simulink model "coif2_7_Level"  (R2021a)
settings: Solver=VariableStepAuto  StartTime=0.0  StopTime=8  RelTol=1e-3
undefined symbols (not defined in the file): lambda2
libraries: dspsigops x15, dspquant2 x1
(part 2 of 4)

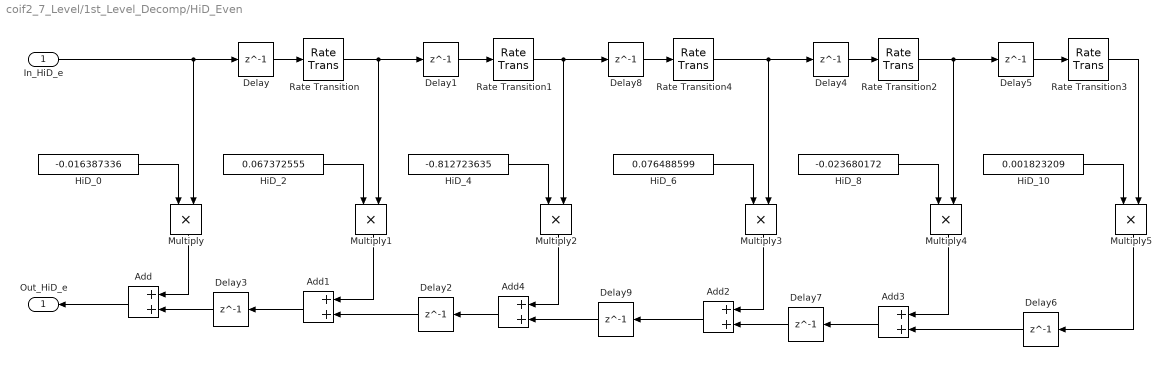
== system coif2_7_Level/1st_Level_Decomp/HiD_Even ==
  In_HiD_e : Inport  OutDataTypeStr=double  SampleTime=1/44100
  Add{,1..4} (5 alike) : Sum  AccumDataTypeStr=double  OutDataTypeStr=double
  Delay{,1..9} (10 alike) : Delay  DelayLength=1  SampleTime=1/44100
  HiD_0 : Constant  Value=-0.016387336  OutDataTypeStr=double  SampleTime=1/44100
  HiD_10 : Constant  Value=0.001823209  OutDataTypeStr=double  SampleTime=1/44100
  HiD_2 : Constant  Value=0.067372555  OutDataTypeStr=double  SampleTime=1/44100
  HiD_4 : Constant  Value=-0.812723635  OutDataTypeStr=double  SampleTime=1/44100
  HiD_6 : Constant  Value=0.076488599  OutDataTypeStr=double  SampleTime=1/44100
  HiD_8 : Constant  Value=-0.023680172  OutDataTypeStr=double  SampleTime=1/44100
  Multiply{,1..5} (6 alike) : Product  OutDataTypeStr=double
  Rate Transition{,1..4} (5 alike) : RateTransition  OutPortSampleTime=1/44100
  Out_HiD_e : Outport  OutDataTypeStr=double  SampleTime=1/44100  VectorParamsAs1DForOutWhenUnconnected=off
  wires:
  In_HiD_e/1 -> Delay/1, Multiply/2
  Delay3/1 -> Add/2
  HiD_2/1 -> Multiply1/1
  Delay/1 -> Rate Transition/1
  Multiply/1 -> Add/1
  Rate Transition/1 -> Delay1/1, Multiply1/2
  HiD_4/1 -> Multiply2/1
  Delay2/1 -> Add1/2
  Multiply1/1 -> Add1/1
  Add1/1 -> Delay3/1
  Rate Transition1/1 -> Delay8/1, Multiply2/2
  Add/1 -> Out_HiD_e/1
  Delay1/1 -> Rate Transition1/1
  HiD_0/1 -> Multiply/1
  HiD_6/1 -> Multiply3/1
  Delay7/1 -> Add2/2
  Delay5/1 -> Rate Transition3/1
  Rate Transition3/1 -> Multiply5/2
  Add3/1 -> Delay7/1
  Multiply3/1 -> Add2/1
  Rate Transition2/1 -> Delay5/1, Multiply4/2
  Delay6/1 -> Add3/2
  Multiply4/1 -> Add3/1
  Multiply5/1 -> Delay6/1
  HiD_10/1 -> Multiply5/1
  Delay4/1 -> Rate Transition2/1
  HiD_8/1 -> Multiply4/1
  Delay8/1 -> Rate Transition4/1
  Rate Transition4/1 -> Multiply3/2, Delay4/1
  Add2/1 -> Delay9/1
  Multiply2/1 -> Add4/1
  Add4/1 -> Delay2/1
  Delay9/1 -> Add4/2

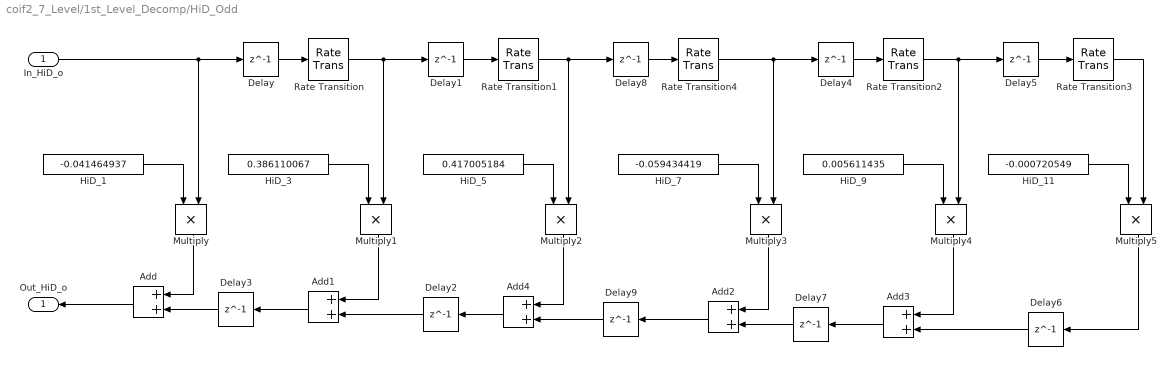
== system coif2_7_Level/1st_Level_Decomp/HiD_Odd ==
  In_HiD_o : Inport  OutDataTypeStr=double  SampleTime=1/44100
  Add{,1..4} (5 alike) : Sum  AccumDataTypeStr=double  OutDataTypeStr=double
  Delay{,1..9} (10 alike) : Delay  DelayLength=1  SampleTime=1/44100
  HiD_1 : Constant  Value=-0.041464937  OutDataTypeStr=double  SampleTime=1/44100
  HiD_11 : Constant  Value=-0.000720549  OutDataTypeStr=double  SampleTime=1/44100
  HiD_3 : Constant  Value=0.386110067  OutDataTypeStr=double  SampleTime=1/44100
  HiD_5 : Constant  Value=0.417005184  OutDataTypeStr=double  SampleTime=1/44100
  HiD_7 : Constant  Value=-0.059434419  OutDataTypeStr=double  SampleTime=1/44100
  HiD_9 : Constant  Value=0.005611435  OutDataTypeStr=double  SampleTime=1/44100
  Multiply{,1..5} (6 alike) : Product  OutDataTypeStr=double
  Rate Transition{,1..4} (5 alike) : RateTransition  OutPortSampleTime=1/44100
  Out_HiD_o : Outport  OutDataTypeStr=double  SampleTime=1/44100  VectorParamsAs1DForOutWhenUnconnected=off
  wires:
  Add/1 -> Out_HiD_o/1
  Add4/1 -> Delay2/1
  Delay8/1 -> Rate Transition4/1
  Rate Transition4/1 -> Multiply3/2, Delay4/1
  HiD_7/1 -> Multiply3/1
  Add2/1 -> Delay9/1
  Delay1/1 -> Rate Transition1/1
  Delay2/1 -> Add1/2
  Delay6/1 -> Add3/2
  HiD_9/1 -> Multiply4/1
  Add3/1 -> Delay7/1
  Multiply3/1 -> Add2/1
  Multiply5/1 -> Delay6/1
  Delay7/1 -> Add2/2
  HiD_3/1 -> Multiply1/1
  Multiply4/1 -> Add3/1
  Rate Transition3/1 -> Multiply5/2
  HiD_1/1 -> Multiply/1
  HiD_11/1 -> Multiply5/1
  Delay4/1 -> Rate Transition2/1
  Rate Transition2/1 -> Delay5/1, Multiply4/2
  Multiply2/1 -> Add4/1
  Delay/1 -> Rate Transition/1
  Rate Transition/1 -> Delay1/1, Multiply1/2
  Delay5/1 -> Rate Transition3/1
  Delay9/1 -> Add4/2
  Multiply1/1 -> Add1/1
  Rate Transition1/1 -> Delay8/1, Multiply2/2
  Multiply/1 -> Add/1
  Add1/1 -> Delay3/1
  Delay3/1 -> Add/2
  In_HiD_o/1 -> Delay/1, Multiply/2
  HiD_5/1 -> Multiply2/1

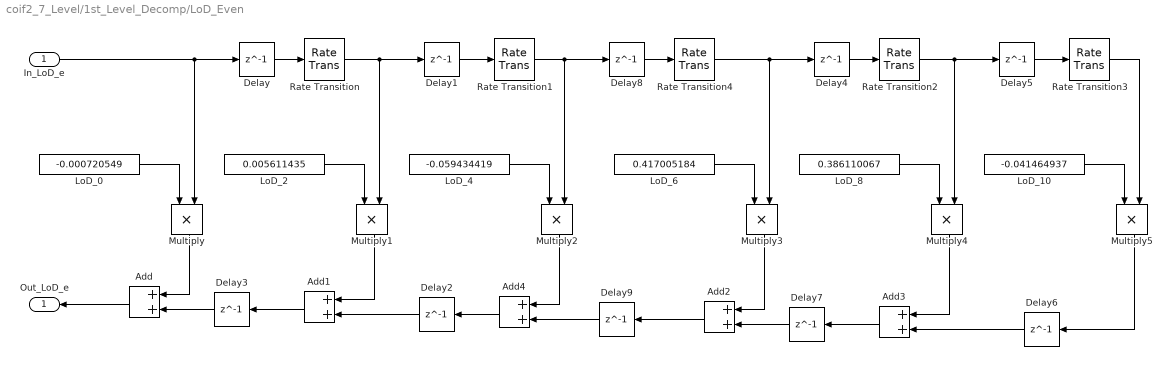
== system coif2_7_Level/1st_Level_Decomp/LoD_Even ==
  In_LoD_e : Inport  OutDataTypeStr=double  SampleTime=1/44100
  Add{,1..4} (5 alike) : Sum  AccumDataTypeStr=double  OutDataTypeStr=double
  Delay{,1..9} (10 alike) : Delay  DelayLength=1  SampleTime=1/44100
  LoD_0 : Constant  Value=-0.000720549  OutDataTypeStr=double  SampleTime=1/44100
  LoD_10 : Constant  Value=-0.041464937  OutDataTypeStr=double  SampleTime=1/44100
  LoD_2 : Constant  Value=0.005611435  OutDataTypeStr=double  SampleTime=1/44100
  LoD_4 : Constant  Value=-0.059434419  OutDataTypeStr=double  SampleTime=1/44100
  LoD_6 : Constant  Value=0.417005184  OutDataTypeStr=double  SampleTime=1/44100
  LoD_8 : Constant  Value=0.386110067  OutDataTypeStr=double  SampleTime=1/44100
  Multiply{,1..5} (6 alike) : Product  OutDataTypeStr=double
  Rate Transition{,1..4} (5 alike) : RateTransition  OutPortSampleTime=1/44100
  Out_LoD_e : Outport  OutDataTypeStr=double  SampleTime=1/44100  VectorParamsAs1DForOutWhenUnconnected=off
  wires:
  Delay3/1 -> Add/2
  Rate Transition1/1 -> Delay8/1, Multiply2/2
  Add/1 -> Out_LoD_e/1
  Add1/1 -> Delay3/1
  Multiply/1 -> Add/1
  In_LoD_e/1 -> Delay/1, Multiply/2
  Rate Transition/1 -> Delay1/1, Multiply1/2
  LoD_4/1 -> Multiply2/1
  Delay/1 -> Rate Transition/1
  Delay9/1 -> Add4/2
  Multiply1/1 -> Add1/1
  Multiply2/1 -> Add4/1
  LoD_2/1 -> Multiply1/1
  Delay4/1 -> Rate Transition2/1
  Multiply5/1 -> Delay6/1
  Multiply4/1 -> Add3/1
  Rate Transition2/1 -> Delay5/1, Multiply4/2
  LoD_10/1 -> Multiply5/1
  Delay2/1 -> Add1/2
  Delay5/1 -> Rate Transition3/1
  Multiply3/1 -> Add2/1
  LoD_8/1 -> Multiply4/1
  Delay7/1 -> Add2/2
  Rate Transition3/1 -> Multiply5/2
  Delay6/1 -> Add3/2
  Add3/1 -> Delay7/1
  LoD_6/1 -> Multiply3/1
  LoD_0/1 -> Multiply/1
  Add2/1 -> Delay9/1
  Delay8/1 -> Rate Transition4/1
  Rate Transition4/1 -> Multiply3/2, Delay4/1
  Delay1/1 -> Rate Transition1/1
  Add4/1 -> Delay2/1

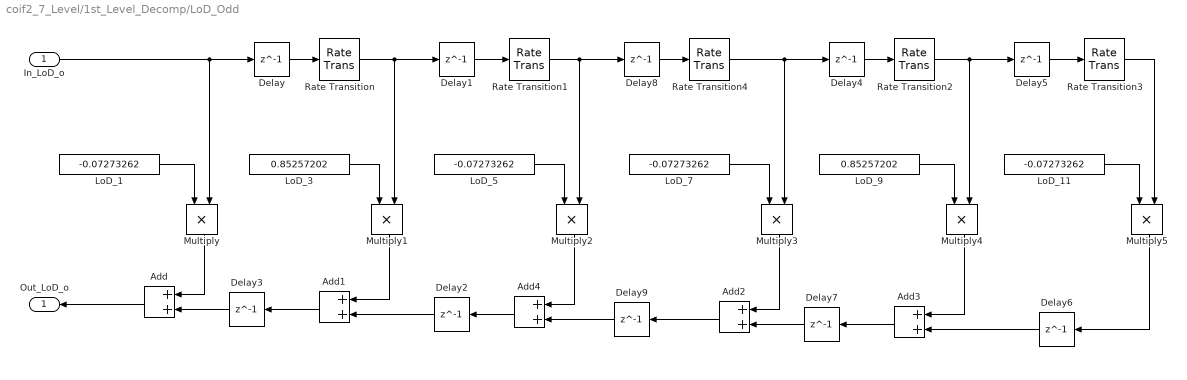
== system coif2_7_Level/1st_Level_Decomp/LoD_Odd ==
  In_LoD_o : Inport  OutDataTypeStr=double  SampleTime=1/44100
  Add{,1..4} (5 alike) : Sum  AccumDataTypeStr=double  OutDataTypeStr=double
  Delay{,1..9} (10 alike) : Delay  DelayLength=1  SampleTime=1/44100
  LoD_{1,5,7,11} (4 alike) : Constant  Value=-0.07273262  OutDataTypeStr=double  SampleTime=1/44100
  LoD_3 : Constant  Value=0.85257202  OutDataTypeStr=double  SampleTime=1/44100
  LoD_9 : Constant  Value=0.85257202  OutDataTypeStr=double  SampleTime=1/44100
  Multiply{,1..5} (6 alike) : Product  OutDataTypeStr=double
  Rate Transition{,1..4} (5 alike) : RateTransition  OutPortSampleTime=1/44100
  Out_LoD_o : Outport  OutDataTypeStr=double  SampleTime=1/44100  VectorParamsAs1DForOutWhenUnconnected=off
  wires:
  LoD_9/1 -> Multiply4/1
  Add3/1 -> Delay7/1
  Rate Transition4/1 -> Multiply3/2, Delay4/1
  Delay2/1 -> Add1/2
  Delay1/1 -> Rate Transition1/1
  Delay8/1 -> Rate Transition4/1
  LoD_5/1 -> Multiply2/1
  Add4/1 -> Delay2/1
  LoD_11/1 -> Multiply5/1
  LoD_1/1 -> Multiply/1
  Multiply3/1 -> Add2/1
  LoD_3/1 -> Multiply1/1
  In_LoD_o/1 -> Delay/1, Multiply/2
  Add/1 -> Out_LoD_o/1
  Rate Transition1/1 -> Delay8/1, Multiply2/2
  Multiply1/1 -> Add1/1
  Delay/1 -> Rate Transition/1
  Rate Transition/1 -> Delay1/1, Multiply1/2
  Multiply2/1 -> Add4/1
  LoD_7/1 -> Multiply3/1
  Rate Transition2/1 -> Delay5/1, Multiply4/2
  Delay4/1 -> Rate Transition2/1
  Multiply5/1 -> Delay6/1
  Delay7/1 -> Add2/2
  Rate Transition3/1 -> Multiply5/2
  Delay3/1 -> Add/2
  Delay5/1 -> Rate Transition3/1
  Add2/1 -> Delay9/1
  Add1/1 -> Delay3/1
  Delay9/1 -> Add4/2
  Delay6/1 -> Add3/2
  Multiply4/1 -> Add3/1
  Multiply/1 -> Add/1

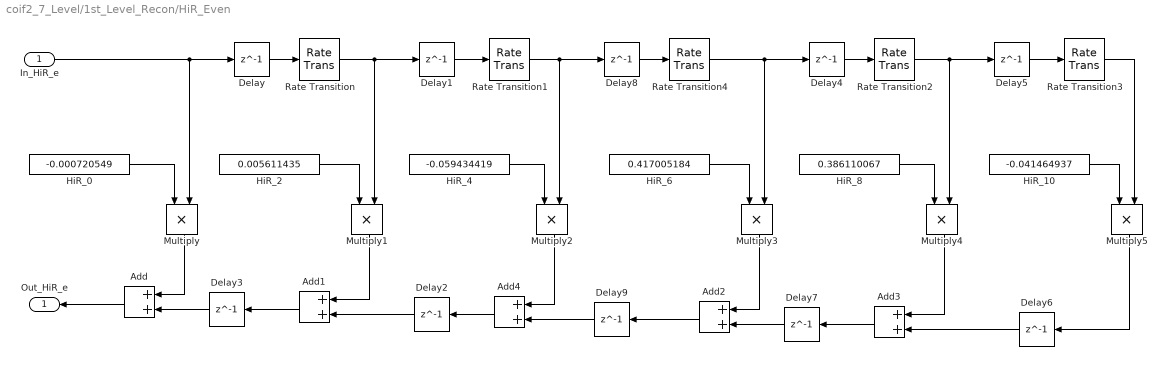
== system coif2_7_Level/1st_Level_Recon/HiR_Even ==
  In_HiR_e : Inport  OutDataTypeStr=double  SampleTime=1/44100
  Add{,1..4} (5 alike) : Sum  AccumDataTypeStr=double  OutDataTypeStr=double
  Delay{,1..9} (10 alike) : Delay  DelayLength=1  SampleTime=1/44100
  HiR_0 : Constant  Value=-0.000720549  OutDataTypeStr=double  SampleTime=1/44100
  HiR_10 : Constant  Value=-0.041464937  OutDataTypeStr=double  SampleTime=1/44100
  HiR_2 : Constant  Value=0.005611435  OutDataTypeStr=double  SampleTime=1/44100
  HiR_4 : Constant  Value=-0.059434419  OutDataTypeStr=double  SampleTime=1/44100
  HiR_6 : Constant  Value=0.417005184  OutDataTypeStr=double  SampleTime=1/44100
  HiR_8 : Constant  Value=0.386110067  OutDataTypeStr=double  SampleTime=1/44100
  Multiply{,1..5} (6 alike) : Product  OutDataTypeStr=double
  Rate Transition{,1..4} (5 alike) : RateTransition  OutPortSampleTime=1/44100
  Out_HiR_e : Outport  OutDataTypeStr=double  SampleTime=1/44100  VectorParamsAs1DForOutWhenUnconnected=off
  wires:
  Multiply1/1 -> Add1/1
  Delay4/1 -> Rate Transition2/1
  Add4/1 -> Delay2/1
  Delay9/1 -> Add4/2
  Rate Transition4/1 -> Multiply3/2, Delay4/1
  Rate Transition3/1 -> Multiply5/2
  Add1/1 -> Delay3/1
  Add3/1 -> Delay7/1
  Delay8/1 -> Rate Transition4/1
  Multiply5/1 -> Delay6/1
  Add2/1 -> Delay9/1
  Multiply4/1 -> Add3/1
  HiR_8/1 -> Multiply4/1
  Delay6/1 -> Add3/2
  Rate Transition1/1 -> Delay8/1, Multiply2/2
  In_HiR_e/1 -> Delay/1, Multiply/2
  HiR_0/1 -> Multiply/1
  Multiply2/1 -> Add4/1
  Delay7/1 -> Add2/2
  Rate Transition2/1 -> Delay5/1, Multiply4/2
  Add/1 -> Out_HiR_e/1
  Multiply3/1 -> Add2/1
  HiR_6/1 -> Multiply3/1
  Multiply/1 -> Add/1
  HiR_4/1 -> Multiply2/1
  Delay2/1 -> Add1/2
  Delay5/1 -> Rate Transition3/1
  Delay3/1 -> Add/2
  Delay1/1 -> Rate Transition1/1
  HiR_2/1 -> Multiply1/1
  Rate Transition/1 -> Delay1/1, Multiply1/2
  Delay/1 -> Rate Transition/1
  HiR_10/1 -> Multiply5/1

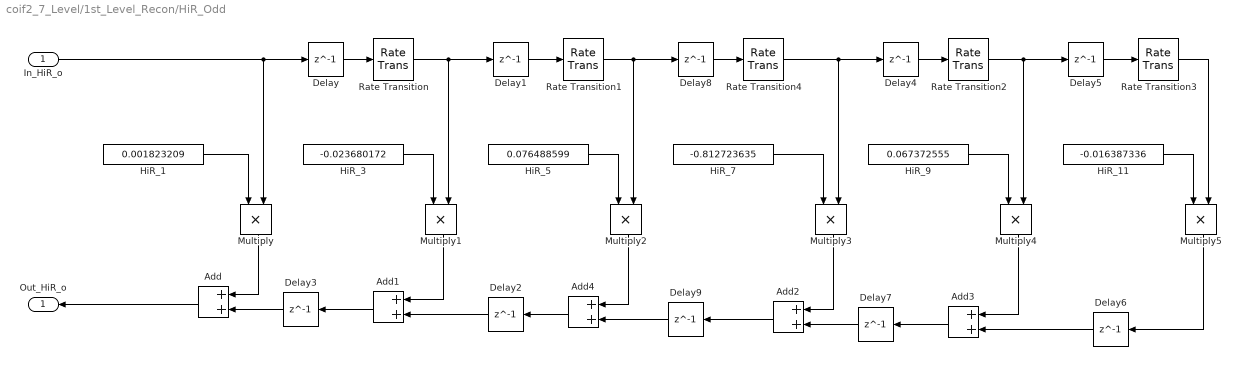
== system coif2_7_Level/1st_Level_Recon/HiR_Odd ==
  In_HiR_o : Inport  OutDataTypeStr=double  SampleTime=1/44100
  Add{,1..4} (5 alike) : Sum  AccumDataTypeStr=double  OutDataTypeStr=double
  Delay{,1..9} (10 alike) : Delay  DelayLength=1  SampleTime=1/44100
  HiR_1 : Constant  Value=0.001823209  OutDataTypeStr=double  SampleTime=1/44100
  HiR_11 : Constant  Value=-0.016387336  OutDataTypeStr=double  SampleTime=1/44100
  HiR_3 : Constant  Value=-0.023680172  OutDataTypeStr=double  SampleTime=1/44100
  HiR_5 : Constant  Value=0.076488599  OutDataTypeStr=double  SampleTime=1/44100
  HiR_7 : Constant  Value=-0.812723635  OutDataTypeStr=double  SampleTime=1/44100
  HiR_9 : Constant  Value=0.067372555  OutDataTypeStr=double  SampleTime=1/44100
  Multiply{,1..5} (6 alike) : Product  OutDataTypeStr=double
  Rate Transition{,1..4} (5 alike) : RateTransition  OutPortSampleTime=1/44100
  Out_HiR_o : Outport  OutDataTypeStr=double  SampleTime=1/44100  VectorParamsAs1DForOutWhenUnconnected=off
  wires:
  HiR_9/1 -> Multiply4/1
  Add2/1 -> Delay9/1
  Rate Transition/1 -> Delay1/1, Multiply1/2
  HiR_7/1 -> Multiply3/1
  Multiply2/1 -> Add4/1
  Rate Transition2/1 -> Delay5/1, Multiply4/2
  Rate Transition4/1 -> Multiply3/2, Delay4/1
  HiR_5/1 -> Multiply2/1
  Multiply5/1 -> Delay6/1
  HiR_11/1 -> Multiply5/1
  Multiply1/1 -> Add1/1
  Delay5/1 -> Rate Transition3/1
  Add1/1 -> Delay3/1
  Multiply/1 -> Add/1
  Delay7/1 -> Add2/2
  Delay2/1 -> Add1/2
  Delay9/1 -> Add4/2
  Delay4/1 -> Rate Transition2/1
  Delay3/1 -> Add/2
  Multiply3/1 -> Add2/1
  Delay8/1 -> Rate Transition4/1
  Rate Transition3/1 -> Multiply5/2
  Delay1/1 -> Rate Transition1/1
  Delay6/1 -> Add3/2
  Add4/1 -> Delay2/1
  Rate Transition1/1 -> Delay8/1, Multiply2/2
  Add/1 -> Out_HiR_o/1
  Add3/1 -> Delay7/1
  HiR_3/1 -> Multiply1/1
  In_HiR_o/1 -> Multiply/2, Delay/1
  Delay/1 -> Rate Transition/1
  HiR_1/1 -> Multiply/1
  Multiply4/1 -> Add3/1

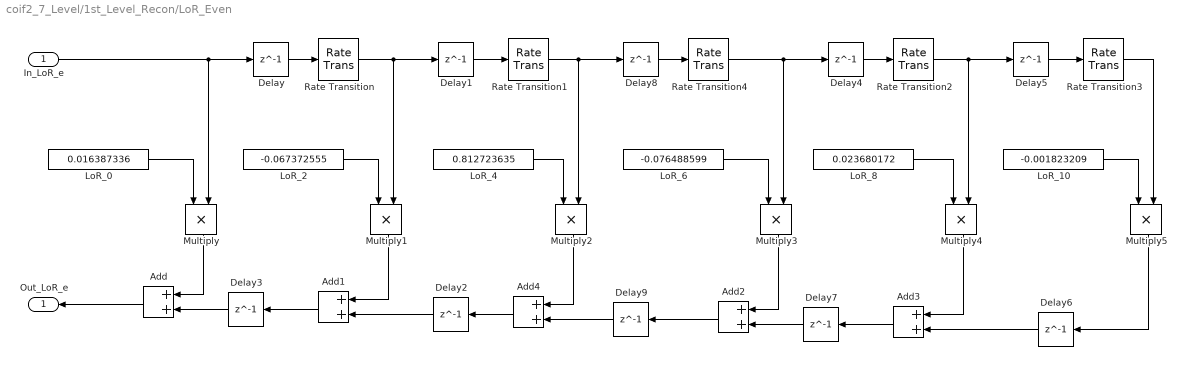
== system coif2_7_Level/1st_Level_Recon/LoR_Even ==
  In_LoR_e : Inport  OutDataTypeStr=double  SampleTime=1/44100
  Add{,1..4} (5 alike) : Sum  AccumDataTypeStr=double  OutDataTypeStr=double
  Delay{,1..9} (10 alike) : Delay  DelayLength=1  SampleTime=1/44100
  LoR_0 : Constant  Value=0.016387336  OutDataTypeStr=double  SampleTime=1/44100
  LoR_10 : Constant  Value=-0.001823209  OutDataTypeStr=double  SampleTime=1/44100
  LoR_2 : Constant  Value=-0.067372555  OutDataTypeStr=double  SampleTime=1/44100
  LoR_4 : Constant  Value=0.812723635  OutDataTypeStr=double  SampleTime=1/44100
  LoR_6 : Constant  Value=-0.076488599  OutDataTypeStr=double  SampleTime=1/44100
  LoR_8 : Constant  Value=0.023680172  OutDataTypeStr=double  SampleTime=1/44100
  Multiply{,1..5} (6 alike) : Product  OutDataTypeStr=double
  Rate Transition{,1..4} (5 alike) : RateTransition  OutPortSampleTime=1/44100
  Out_LoR_e : Outport  OutDataTypeStr=double  SampleTime=1/44100  VectorParamsAs1DForOutWhenUnconnected=off
  wires:
  LoR_4/1 -> Multiply2/1
  LoR_10/1 -> Multiply5/1
  LoR_8/1 -> Multiply4/1
  LoR_0/1 -> Multiply/1
  LoR_2/1 -> Multiply1/1
  Add2/1 -> Delay9/1
  In_LoR_e/1 -> Multiply/2, Delay/1
  Multiply4/1 -> Add3/1
  Delay8/1 -> Rate Transition4/1
  Add3/1 -> Delay7/1
  Rate Transition3/1 -> Multiply5/2
  Add4/1 -> Delay2/1
  Delay4/1 -> Rate Transition2/1
  Multiply1/1 -> Add1/1
  Delay5/1 -> Rate Transition3/1
  Delay2/1 -> Add1/2
  Delay3/1 -> Add/2
  Delay1/1 -> Rate Transition1/1
  Multiply/1 -> Add/1
  Multiply3/1 -> Add2/1
  Delay9/1 -> Add4/2
  Rate Transition2/1 -> Delay5/1, Multiply4/2
  Rate Transition4/1 -> Multiply3/2, Delay4/1
  Add1/1 -> Delay3/1
  LoR_6/1 -> Multiply3/1
  Multiply5/1 -> Delay6/1
  Add/1 -> Out_LoR_e/1
  Rate Transition1/1 -> Delay8/1, Multiply2/2
  Delay6/1 -> Add3/2
  Multiply2/1 -> Add4/1
  Delay7/1 -> Add2/2
  Rate Transition/1 -> Delay1/1, Multiply1/2
  Delay/1 -> Rate Transition/1

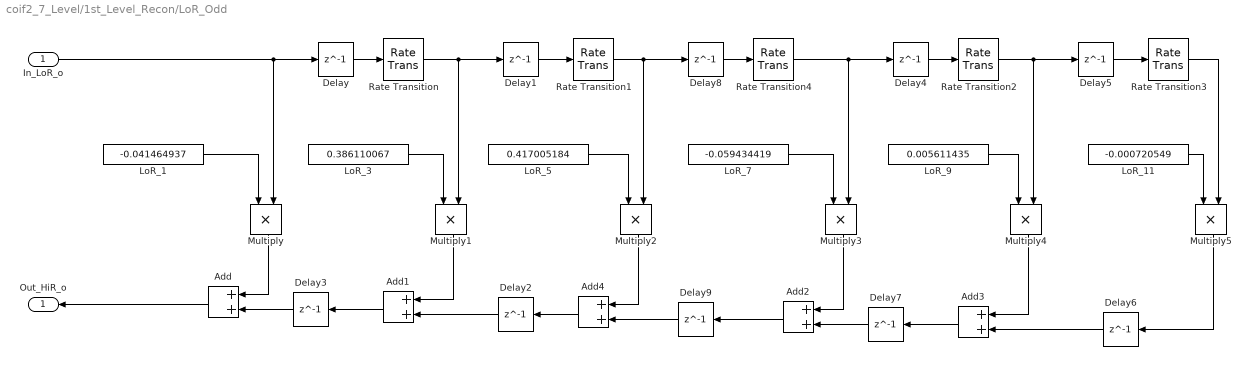
== system coif2_7_Level/1st_Level_Recon/LoR_Odd ==
  In_LoR_o : Inport  OutDataTypeStr=double  SampleTime=1/44100
  Add{,1..4} (5 alike) : Sum  AccumDataTypeStr=double  OutDataTypeStr=double
  Delay{,1..9} (10 alike) : Delay  DelayLength=1  SampleTime=1/44100
  LoR_1 : Constant  Value=-0.041464937  OutDataTypeStr=double  SampleTime=1/44100
  LoR_11 : Constant  Value=-0.000720549  OutDataTypeStr=double  SampleTime=1/44100
  LoR_3 : Constant  Value=0.386110067  OutDataTypeStr=double  SampleTime=1/44100
  LoR_5 : Constant  Value=0.417005184  OutDataTypeStr=double  SampleTime=1/44100
  LoR_7 : Constant  Value=-0.059434419  OutDataTypeStr=double  SampleTime=1/44100
  LoR_9 : Constant  Value=0.005611435  OutDataTypeStr=double  SampleTime=1/44100
  Multiply{,1..5} (6 alike) : Product  OutDataTypeStr=double
  Rate Transition{,1..4} (5 alike) : RateTransition  OutPortSampleTime=1/44100
  Out_HiR_o : Outport  OutDataTypeStr=double  SampleTime=1/44100  VectorParamsAs1DForOutWhenUnconnected=off
  wires:
  LoR_9/1 -> Multiply4/1
  Add2/1 -> Delay9/1
  Rate Transition/1 -> Delay1/1, Multiply1/2
  LoR_7/1 -> Multiply3/1
  Multiply2/1 -> Add4/1
  Rate Transition2/1 -> Delay5/1, Multiply4/2
  Rate Transition4/1 -> Multiply3/2, Delay4/1
  LoR_5/1 -> Multiply2/1
  Multiply5/1 -> Delay6/1
  LoR_11/1 -> Multiply5/1
  Multiply1/1 -> Add1/1
  Delay5/1 -> Rate Transition3/1
  Add1/1 -> Delay3/1
  Multiply/1 -> Add/1
  Delay7/1 -> Add2/2
  Delay2/1 -> Add1/2
  Delay9/1 -> Add4/2
  Delay4/1 -> Rate Transition2/1
  Delay3/1 -> Add/2
  Multiply3/1 -> Add2/1
  Delay8/1 -> Rate Transition4/1
  Rate Transition3/1 -> Multiply5/2
  Delay1/1 -> Rate Transition1/1
  Delay6/1 -> Add3/2
  Add4/1 -> Delay2/1
  Rate Transition1/1 -> Delay8/1, Multiply2/2
  Add/1 -> Out_HiR_o/1
  Add3/1 -> Delay7/1
  LoR_3/1 -> Multiply1/1
  In_LoR_o/1 -> Multiply/2, Delay/1
  Delay/1 -> Rate Transition/1
  LoR_1/1 -> Multiply/1
  Multiply4/1 -> Add3/1

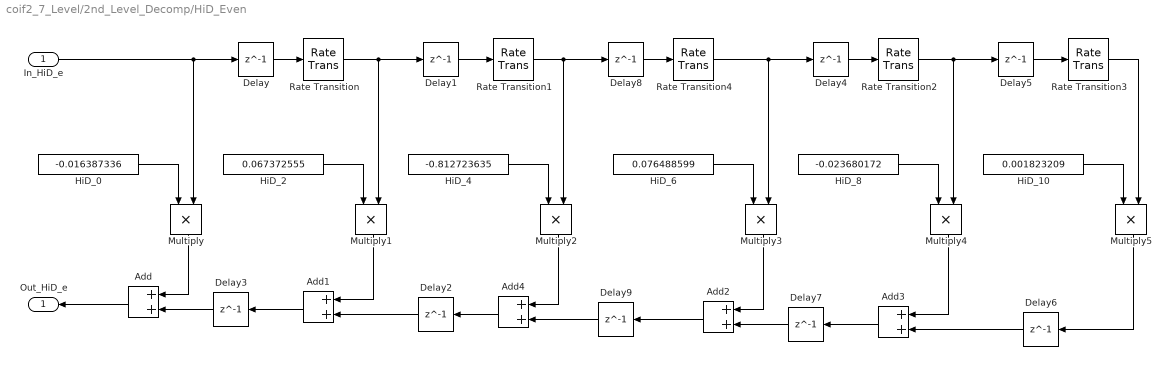
== system coif2_7_Level/2nd_Level_Decomp/HiD_Even ==
  In_HiD_e : Inport  OutDataTypeStr=double  SampleTime=1/44100
  Add{,1..4} (5 alike) : Sum  AccumDataTypeStr=double  OutDataTypeStr=double
  Delay{,1..9} (10 alike) : Delay  DelayLength=1  SampleTime=1/44100
  HiD_0 : Constant  Value=-0.016387336  OutDataTypeStr=double  SampleTime=1/44100
  HiD_10 : Constant  Value=0.001823209  OutDataTypeStr=double  SampleTime=1/44100
  HiD_2 : Constant  Value=0.067372555  OutDataTypeStr=double  SampleTime=1/44100
  HiD_4 : Constant  Value=-0.812723635  OutDataTypeStr=double  SampleTime=1/44100
  HiD_6 : Constant  Value=0.076488599  OutDataTypeStr=double  SampleTime=1/44100
  HiD_8 : Constant  Value=-0.023680172  OutDataTypeStr=double  SampleTime=1/44100
  Multiply{,1..5} (6 alike) : Product  OutDataTypeStr=double
  Rate Transition{,1..4} (5 alike) : RateTransition  OutPortSampleTime=1/44100
  Out_HiD_e : Outport  OutDataTypeStr=double  SampleTime=1/44100  VectorParamsAs1DForOutWhenUnconnected=off
  wires:
  In_HiD_e/1 -> Delay/1, Multiply/2
  Delay3/1 -> Add/2
  HiD_2/1 -> Multiply1/1
  Delay/1 -> Rate Transition/1
  Multiply/1 -> Add/1
  Rate Transition/1 -> Delay1/1, Multiply1/2
  HiD_4/1 -> Multiply2/1
  Delay2/1 -> Add1/2
  Multiply1/1 -> Add1/1
  Add1/1 -> Delay3/1
  Rate Transition1/1 -> Delay8/1, Multiply2/2
  Add/1 -> Out_HiD_e/1
  Delay1/1 -> Rate Transition1/1
  HiD_0/1 -> Multiply/1
  HiD_6/1 -> Multiply3/1
  Delay7/1 -> Add2/2
  Delay5/1 -> Rate Transition3/1
  Rate Transition3/1 -> Multiply5/2
  Add3/1 -> Delay7/1
  Multiply3/1 -> Add2/1
  Rate Transition2/1 -> Delay5/1, Multiply4/2
  Delay6/1 -> Add3/2
  Multiply4/1 -> Add3/1
  Multiply5/1 -> Delay6/1
  HiD_10/1 -> Multiply5/1
  Delay4/1 -> Rate Transition2/1
  HiD_8/1 -> Multiply4/1
  Delay8/1 -> Rate Transition4/1
  Rate Transition4/1 -> Multiply3/2, Delay4/1
  Add2/1 -> Delay9/1
  Multiply2/1 -> Add4/1
  Add4/1 -> Delay2/1
  Delay9/1 -> Add4/2

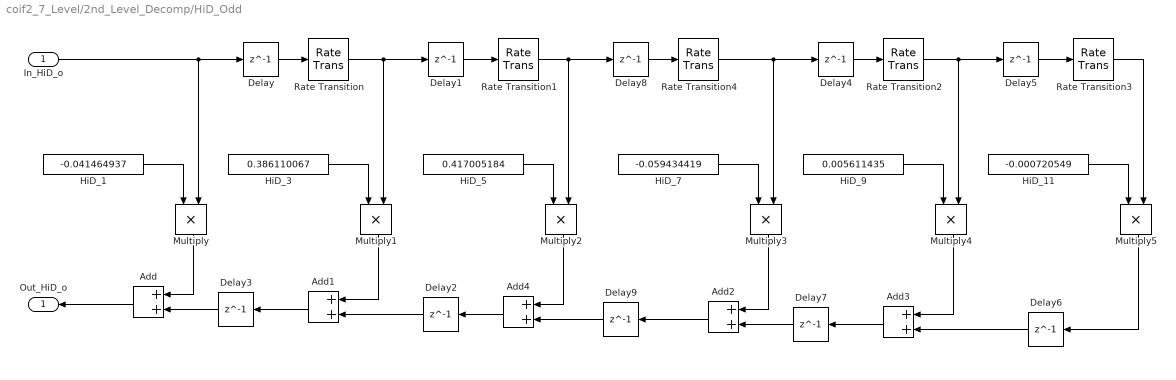
== system coif2_7_Level/2nd_Level_Decomp/HiD_Odd ==
  In_HiD_o : Inport  OutDataTypeStr=double  SampleTime=1/44100
  Add{,1..4} (5 alike) : Sum  AccumDataTypeStr=double  OutDataTypeStr=double
  Delay{,1..9} (10 alike) : Delay  DelayLength=1  SampleTime=1/44100
  HiD_1 : Constant  Value=-0.041464937  OutDataTypeStr=double  SampleTime=1/44100
  HiD_11 : Constant  Value=-0.000720549  OutDataTypeStr=double  SampleTime=1/44100
  HiD_3 : Constant  Value=0.386110067  OutDataTypeStr=double  SampleTime=1/44100
  HiD_5 : Constant  Value=0.417005184  OutDataTypeStr=double  SampleTime=1/44100
  HiD_7 : Constant  Value=-0.059434419  OutDataTypeStr=double  SampleTime=1/44100
  HiD_9 : Constant  Value=0.005611435  OutDataTypeStr=double  SampleTime=1/44100
  Multiply{,1..5} (6 alike) : Product  OutDataTypeStr=double
  Rate Transition{,1..4} (5 alike) : RateTransition  OutPortSampleTime=1/44100
  Out_HiD_o : Outport  OutDataTypeStr=double  SampleTime=1/44100  VectorParamsAs1DForOutWhenUnconnected=off
  wires:
  Add/1 -> Out_HiD_o/1
  Add4/1 -> Delay2/1
  Delay8/1 -> Rate Transition4/1
  Rate Transition4/1 -> Multiply3/2, Delay4/1
  HiD_7/1 -> Multiply3/1
  Add2/1 -> Delay9/1
  Delay1/1 -> Rate Transition1/1
  Delay2/1 -> Add1/2
  Delay6/1 -> Add3/2
  HiD_9/1 -> Multiply4/1
  Add3/1 -> Delay7/1
  Multiply3/1 -> Add2/1
  Multiply5/1 -> Delay6/1
  Delay7/1 -> Add2/2
  HiD_3/1 -> Multiply1/1
  Multiply4/1 -> Add3/1
  Rate Transition3/1 -> Multiply5/2
  HiD_1/1 -> Multiply/1
  HiD_11/1 -> Multiply5/1
  Delay4/1 -> Rate Transition2/1
  Rate Transition2/1 -> Delay5/1, Multiply4/2
  Multiply2/1 -> Add4/1
  Delay/1 -> Rate Transition/1
  Rate Transition/1 -> Delay1/1, Multiply1/2
  Delay5/1 -> Rate Transition3/1
  Delay9/1 -> Add4/2
  Multiply1/1 -> Add1/1
  Rate Transition1/1 -> Delay8/1, Multiply2/2
  Multiply/1 -> Add/1
  Add1/1 -> Delay3/1
  Delay3/1 -> Add/2
  In_HiD_o/1 -> Delay/1, Multiply/2
  HiD_5/1 -> Multiply2/1

== system coif2_7_Level/2nd_Level_Decomp/LoD_Even ==
  In_LoD_e : Inport  OutDataTypeStr=double  SampleTime=1/44100
  Add{,1..4} (5 alike) : Sum  AccumDataTypeStr=double  OutDataTypeStr=double
  Delay{,1..9} (10 alike) : Delay  DelayLength=1  SampleTime=1/44100
  LoD_0 : Constant  Value=-0.000720549  OutDataTypeStr=double  SampleTime=1/44100
  LoD_10 : Constant  Value=-0.041464937  OutDataTypeStr=double  SampleTime=1/44100
  LoD_2 : Constant  Value=0.005611435  OutDataTypeStr=double  SampleTime=1/44100
  LoD_4 : Constant  Value=-0.059434419  OutDataTypeStr=double  SampleTime=1/44100
  LoD_6 : Constant  Value=0.417005184  OutDataTypeStr=double  SampleTime=1/44100
  LoD_8 : Constant  Value=0.386110067  OutDataTypeStr=double  SampleTime=1/44100
  Multiply{,1..5} (6 alike) : Product  OutDataTypeStr=double
  Rate Transition{,1..4} (5 alike) : RateTransition  OutPortSampleTime=1/44100
  Out_LoD_e : Outport  OutDataTypeStr=double  SampleTime=1/44100  VectorParamsAs1DForOutWhenUnconnected=off
  wires:
  Delay3/1 -> Add/2
  Rate Transition1/1 -> Delay8/1, Multiply2/2
  Add/1 -> Out_LoD_e/1
  Add1/1 -> Delay3/1
  Multiply/1 -> Add/1
  In_LoD_e/1 -> Delay/1, Multiply/2
  Rate Transition/1 -> Delay1/1, Multiply1/2
  LoD_4/1 -> Multiply2/1
  Delay/1 -> Rate Transition/1
  Delay9/1 -> Add4/2
  Multiply1/1 -> Add1/1
  Multiply2/1 -> Add4/1
  LoD_2/1 -> Multiply1/1
  Delay4/1 -> Rate Transition2/1
  Multiply5/1 -> Delay6/1
  Multiply4/1 -> Add3/1
  Rate Transition2/1 -> Delay5/1, Multiply4/2
  LoD_10/1 -> Multiply5/1
  Delay2/1 -> Add1/2
  Delay5/1 -> Rate Transition3/1
  Multiply3/1 -> Add2/1
  LoD_8/1 -> Multiply4/1
  Delay7/1 -> Add2/2
  Rate Transition3/1 -> Multiply5/2
  Delay6/1 -> Add3/2
  Add3/1 -> Delay7/1
  LoD_6/1 -> Multiply3/1
  LoD_0/1 -> Multiply/1
  Add2/1 -> Delay9/1
  Delay8/1 -> Rate Transition4/1
  Rate Transition4/1 -> Multiply3/2, Delay4/1
  Delay1/1 -> Rate Transition1/1
  Add4/1 -> Delay2/1

== system coif2_7_Level/2nd_Level_Decomp/LoD_Odd ==
  In_LoD_o : Inport  OutDataTypeStr=double  SampleTime=1/44100
  Add{,1..4} (5 alike) : Sum  AccumDataTypeStr=double  OutDataTypeStr=double
  Delay{,1..9} (10 alike) : Delay  DelayLength=1  SampleTime=1/44100
  LoD_{1,5,7,11} (4 alike) : Constant  Value=-0.07273262  OutDataTypeStr=double  SampleTime=1/44100
  LoD_3 : Constant  Value=0.85257202  OutDataTypeStr=double  SampleTime=1/44100
  LoD_9 : Constant  Value=0.85257202  OutDataTypeStr=double  SampleTime=1/44100
  Multiply{,1..5} (6 alike) : Product  OutDataTypeStr=double
  Rate Transition{,1..4} (5 alike) : RateTransition  OutPortSampleTime=1/44100
  Out_LoD_o : Outport  OutDataTypeStr=double  SampleTime=1/44100  VectorParamsAs1DForOutWhenUnconnected=off
  wires:
  LoD_9/1 -> Multiply4/1
  Add3/1 -> Delay7/1
  Rate Transition4/1 -> Multiply3/2, Delay4/1
  Delay2/1 -> Add1/2
  Delay1/1 -> Rate Transition1/1
  Delay8/1 -> Rate Transition4/1
  LoD_5/1 -> Multiply2/1
  Add4/1 -> Delay2/1
  LoD_11/1 -> Multiply5/1
  LoD_1/1 -> Multiply/1
  Multiply3/1 -> Add2/1
  LoD_3/1 -> Multiply1/1
  In_LoD_o/1 -> Delay/1, Multiply/2
  Add/1 -> Out_LoD_o/1
  Rate Transition1/1 -> Delay8/1, Multiply2/2
  Multiply1/1 -> Add1/1
  Delay/1 -> Rate Transition/1
  Rate Transition/1 -> Delay1/1, Multiply1/2
  Multiply2/1 -> Add4/1
  LoD_7/1 -> Multiply3/1
  Rate Transition2/1 -> Delay5/1, Multiply4/2
  Delay4/1 -> Rate Transition2/1
  Multiply5/1 -> Delay6/1
  Delay7/1 -> Add2/2
  Rate Transition3/1 -> Multiply5/2
  Delay3/1 -> Add/2
  Delay5/1 -> Rate Transition3/1
  Add2/1 -> Delay9/1
  Add1/1 -> Delay3/1
  Delay9/1 -> Add4/2
  Delay6/1 -> Add3/2
  Multiply4/1 -> Add3/1
  Multiply/1 -> Add/1

== system coif2_7_Level/2nd_Level_Recon/HiR_Even ==
  In_HiR_e : Inport  OutDataTypeStr=double  SampleTime=1/44100
  Add{,1..4} (5 alike) : Sum  AccumDataTypeStr=double  OutDataTypeStr=double
  Delay{,1..9} (10 alike) : Delay  DelayLength=1  SampleTime=1/44100
  HiR_0 : Constant  Value=-0.000720549  OutDataTypeStr=double  SampleTime=1/44100
  HiR_10 : Constant  Value=-0.041464937  OutDataTypeStr=double  SampleTime=1/44100
  HiR_2 : Constant  Value=0.005611435  OutDataTypeStr=double  SampleTime=1/44100
  HiR_4 : Constant  Value=-0.059434419  OutDataTypeStr=double  SampleTime=1/44100
  HiR_6 : Constant  Value=0.417005184  OutDataTypeStr=double  SampleTime=1/44100
  HiR_8 : Constant  Value=0.386110067  OutDataTypeStr=double  SampleTime=1/44100
  Multiply{,1..5} (6 alike) : Product  OutDataTypeStr=double
  Rate Transition{,1..4} (5 alike) : RateTransition  OutPortSampleTime=1/44100
  Out_HiR_e : Outport  OutDataTypeStr=double  SampleTime=1/44100  VectorParamsAs1DForOutWhenUnconnected=off
  wires:
  Multiply1/1 -> Add1/1
  Delay4/1 -> Rate Transition2/1
  Add4/1 -> Delay2/1
  Delay9/1 -> Add4/2
  Rate Transition4/1 -> Multiply3/2, Delay4/1
  Rate Transition3/1 -> Multiply5/2
  Add1/1 -> Delay3/1
  Add3/1 -> Delay7/1
  Delay8/1 -> Rate Transition4/1
  Multiply5/1 -> Delay6/1
  Add2/1 -> Delay9/1
  Multiply4/1 -> Add3/1
  HiR_8/1 -> Multiply4/1
  Delay6/1 -> Add3/2
  Rate Transition1/1 -> Delay8/1, Multiply2/2
  In_HiR_e/1 -> Delay/1, Multiply/2
  HiR_0/1 -> Multiply/1
  Multiply2/1 -> Add4/1
  Delay7/1 -> Add2/2
  Rate Transition2/1 -> Delay5/1, Multiply4/2
  Add/1 -> Out_HiR_e/1
  Multiply3/1 -> Add2/1
  HiR_6/1 -> Multiply3/1
  Multiply/1 -> Add/1
  HiR_4/1 -> Multiply2/1
  Delay2/1 -> Add1/2
  Delay5/1 -> Rate Transition3/1
  Delay3/1 -> Add/2
  Delay1/1 -> Rate Transition1/1
  HiR_2/1 -> Multiply1/1
  Rate Transition/1 -> Delay1/1, Multiply1/2
  Delay/1 -> Rate Transition/1
  HiR_10/1 -> Multiply5/1

== system coif2_7_Level/2nd_Level_Recon/HiR_Odd ==
  In_HiR_o : Inport  OutDataTypeStr=double  SampleTime=1/44100
  Add{,1..4} (5 alike) : Sum  AccumDataTypeStr=double  OutDataTypeStr=double
  Delay{,1..9} (10 alike) : Delay  DelayLength=1  SampleTime=1/44100
  HiR_1 : Constant  Value=0.001823209  OutDataTypeStr=double  SampleTime=1/44100
  HiR_11 : Constant  Value=-0.016387336  OutDataTypeStr=double  SampleTime=1/44100
  HiR_3 : Constant  Value=-0.023680172  OutDataTypeStr=double  SampleTime=1/44100
  HiR_5 : Constant  Value=0.076488599  OutDataTypeStr=double  SampleTime=1/44100
  HiR_7 : Constant  Value=-0.812723635  OutDataTypeStr=double  SampleTime=1/44100
  HiR_9 : Constant  Value=0.067372555  OutDataTypeStr=double  SampleTime=1/44100
  Multiply{,1..5} (6 alike) : Product  OutDataTypeStr=double
  Rate Transition{,1..4} (5 alike) : RateTransition  OutPortSampleTime=1/44100
  Out_HiR_o : Outport  OutDataTypeStr=double  SampleTime=1/44100  VectorParamsAs1DForOutWhenUnconnected=off
  wires:
  HiR_9/1 -> Multiply4/1
  Add2/1 -> Delay9/1
  Rate Transition/1 -> Delay1/1, Multiply1/2
  HiR_7/1 -> Multiply3/1
  Multiply2/1 -> Add4/1
  Rate Transition2/1 -> Delay5/1, Multiply4/2
  Rate Transition4/1 -> Multiply3/2, Delay4/1
  HiR_5/1 -> Multiply2/1
  Multiply5/1 -> Delay6/1
  HiR_11/1 -> Multiply5/1
  Multiply1/1 -> Add1/1
  Delay5/1 -> Rate Transition3/1
  Add1/1 -> Delay3/1
  Multiply/1 -> Add/1
  Delay7/1 -> Add2/2
  Delay2/1 -> Add1/2
  Delay9/1 -> Add4/2
  Delay4/1 -> Rate Transition2/1
  Delay3/1 -> Add/2
  Multiply3/1 -> Add2/1
  Delay8/1 -> Rate Transition4/1
  Rate Transition3/1 -> Multiply5/2
  Delay1/1 -> Rate Transition1/1
  Delay6/1 -> Add3/2
  Add4/1 -> Delay2/1
  Rate Transition1/1 -> Delay8/1, Multiply2/2
  Add/1 -> Out_HiR_o/1
  Add3/1 -> Delay7/1
  HiR_3/1 -> Multiply1/1
  In_HiR_o/1 -> Multiply/2, Delay/1
  Delay/1 -> Rate Transition/1
  HiR_1/1 -> Multiply/1
  Multiply4/1 -> Add3/1

== system coif2_7_Level/2nd_Level_Recon/LoR_Even ==
  In_LoR_e : Inport  OutDataTypeStr=double  SampleTime=1/44100
  Add{,1..4} (5 alike) : Sum  AccumDataTypeStr=double  OutDataTypeStr=double
  Delay{,1..9} (10 alike) : Delay  DelayLength=1  SampleTime=1/44100
  LoR_0 : Constant  Value=0.016387336  OutDataTypeStr=double  SampleTime=1/44100
  LoR_10 : Constant  Value=-0.001823209  OutDataTypeStr=double  SampleTime=1/44100
  LoR_2 : Constant  Value=-0.067372555  OutDataTypeStr=double  SampleTime=1/44100
  LoR_4 : Constant  Value=0.812723635  OutDataTypeStr=double  SampleTime=1/44100
  LoR_6 : Constant  Value=-0.076488599  OutDataTypeStr=double  SampleTime=1/44100
  LoR_8 : Constant  Value=0.023680172  OutDataTypeStr=double  SampleTime=1/44100
  Multiply{,1..5} (6 alike) : Product  OutDataTypeStr=double
  Rate Transition{,1..4} (5 alike) : RateTransition  OutPortSampleTime=1/44100
  Out_LoR_e : Outport  OutDataTypeStr=double  SampleTime=1/44100  VectorParamsAs1DForOutWhenUnconnected=off
  wires:
  LoR_4/1 -> Multiply2/1
  LoR_10/1 -> Multiply5/1
  LoR_8/1 -> Multiply4/1
  LoR_0/1 -> Multiply/1
  LoR_2/1 -> Multiply1/1
  Add2/1 -> Delay9/1
  In_LoR_e/1 -> Multiply/2, Delay/1
  Multiply4/1 -> Add3/1
  Delay8/1 -> Rate Transition4/1
  Add3/1 -> Delay7/1
  Rate Transition3/1 -> Multiply5/2
  Add4/1 -> Delay2/1
  Delay4/1 -> Rate Transition2/1
  Multiply1/1 -> Add1/1
  Delay5/1 -> Rate Transition3/1
  Delay2/1 -> Add1/2
  Delay3/1 -> Add/2
  Delay1/1 -> Rate Transition1/1
  Multiply/1 -> Add/1
  Multiply3/1 -> Add2/1
  Delay9/1 -> Add4/2
  Rate Transition2/1 -> Delay5/1, Multiply4/2
  Rate Transition4/1 -> Multiply3/2, Delay4/1
  Add1/1 -> Delay3/1
  LoR_6/1 -> Multiply3/1
  Multiply5/1 -> Delay6/1
  Add/1 -> Out_LoR_e/1
  Rate Transition1/1 -> Delay8/1, Multiply2/2
  Delay6/1 -> Add3/2
  Multiply2/1 -> Add4/1
  Delay7/1 -> Add2/2
  Rate Transition/1 -> Delay1/1, Multiply1/2
  Delay/1 -> Rate Transition/1

== system coif2_7_Level/2nd_Level_Recon/LoR_Odd ==
  In_LoR_o : Inport  OutDataTypeStr=double  SampleTime=1/44100
  Add{,1..4} (5 alike) : Sum  AccumDataTypeStr=double  OutDataTypeStr=double
  Delay{,1..9} (10 alike) : Delay  DelayLength=1  SampleTime=1/44100
  LoR_1 : Constant  Value=-0.041464937  OutDataTypeStr=double  SampleTime=1/44100
  LoR_11 : Constant  Value=-0.000720549  OutDataTypeStr=double  SampleTime=1/44100
  LoR_3 : Constant  Value=0.386110067  OutDataTypeStr=double  SampleTime=1/44100
  LoR_5 : Constant  Value=0.417005184  OutDataTypeStr=double  SampleTime=1/44100
  LoR_7 : Constant  Value=-0.059434419  OutDataTypeStr=double  SampleTime=1/44100
  LoR_9 : Constant  Value=0.005611435  OutDataTypeStr=double  SampleTime=1/44100
  Multiply{,1..5} (6 alike) : Product  OutDataTypeStr=double
  Rate Transition{,1..4} (5 alike) : RateTransition  OutPortSampleTime=1/44100
  Out_HiR_o : Outport  OutDataTypeStr=double  SampleTime=1/44100  VectorParamsAs1DForOutWhenUnconnected=off
  wires:
  LoR_9/1 -> Multiply4/1
  Add2/1 -> Delay9/1
  Rate Transition/1 -> Delay1/1, Multiply1/2
  LoR_7/1 -> Multiply3/1
  Multiply2/1 -> Add4/1
  Rate Transition2/1 -> Delay5/1, Multiply4/2
  Rate Transition4/1 -> Multiply3/2, Delay4/1
  LoR_5/1 -> Multiply2/1
  Multiply5/1 -> Delay6/1
  LoR_11/1 -> Multiply5/1
  Multiply1/1 -> Add1/1
  Delay5/1 -> Rate Transition3/1
  Add1/1 -> Delay3/1
  Multiply/1 -> Add/1
  Delay7/1 -> Add2/2
  Delay2/1 -> Add1/2
  Delay9/1 -> Add4/2
  Delay4/1 -> Rate Transition2/1
  Delay3/1 -> Add/2
  Multiply3/1 -> Add2/1
  Delay8/1 -> Rate Transition4/1
  Rate Transition3/1 -> Multiply5/2
  Delay1/1 -> Rate Transition1/1
  Delay6/1 -> Add3/2
  Add4/1 -> Delay2/1
  Rate Transition1/1 -> Delay8/1, Multiply2/2
  Add/1 -> Out_HiR_o/1
  Add3/1 -> Delay7/1
  LoR_3/1 -> Multiply1/1
  In_LoR_o/1 -> Multiply/2, Delay/1
  Delay/1 -> Rate Transition/1
  LoR_1/1 -> Multiply/1
  Multiply4/1 -> Add3/1

== system coif2_7_Level/3rd_Level_Decomp/HiD_Even ==
  In_HiD_e : Inport  OutDataTypeStr=double  SampleTime=1/44100
  Add{,1..4} (5 alike) : Sum  AccumDataTypeStr=double  OutDataTypeStr=double
  Delay{,1..9} (10 alike) : Delay  DelayLength=1  SampleTime=1/44100
  HiD_0 : Constant  Value=-0.016387336  OutDataTypeStr=double  SampleTime=1/44100
  HiD_10 : Constant  Value=0.001823209  OutDataTypeStr=double  SampleTime=1/44100
  HiD_2 : Constant  Value=0.067372555  OutDataTypeStr=double  SampleTime=1/44100
  HiD_4 : Constant  Value=-0.812723635  OutDataTypeStr=double  SampleTime=1/44100
  HiD_6 : Constant  Value=0.076488599  OutDataTypeStr=double  SampleTime=1/44100
  HiD_8 : Constant  Value=-0.023680172  OutDataTypeStr=double  SampleTime=1/44100
  Multiply{,1..5} (6 alike) : Product  OutDataTypeStr=double
  Rate Transition{,1..4} (5 alike) : RateTransition  OutPortSampleTime=1/44100
  Out_HiD_e : Outport  OutDataTypeStr=double  SampleTime=1/44100  VectorParamsAs1DForOutWhenUnconnected=off
  wires:
  In_HiD_e/1 -> Delay/1, Multiply/2
  Delay3/1 -> Add/2
  HiD_2/1 -> Multiply1/1
  Delay/1 -> Rate Transition/1
  Multiply/1 -> Add/1
  Rate Transition/1 -> Delay1/1, Multiply1/2
  HiD_4/1 -> Multiply2/1
  Delay2/1 -> Add1/2
  Multiply1/1 -> Add1/1
  Add1/1 -> Delay3/1
  Rate Transition1/1 -> Delay8/1, Multiply2/2
  Add/1 -> Out_HiD_e/1
  Delay1/1 -> Rate Transition1/1
  HiD_0/1 -> Multiply/1
  HiD_6/1 -> Multiply3/1
  Delay7/1 -> Add2/2
  Delay5/1 -> Rate Transition3/1
  Rate Transition3/1 -> Multiply5/2
  Add3/1 -> Delay7/1
  Multiply3/1 -> Add2/1
  Rate Transition2/1 -> Delay5/1, Multiply4/2
  Delay6/1 -> Add3/2
  Multiply4/1 -> Add3/1
  Multiply5/1 -> Delay6/1
  HiD_10/1 -> Multiply5/1
  Delay4/1 -> Rate Transition2/1
  HiD_8/1 -> Multiply4/1
  Delay8/1 -> Rate Transition4/1
  Rate Transition4/1 -> Multiply3/2, Delay4/1
  Add2/1 -> Delay9/1
  Multiply2/1 -> Add4/1
  Add4/1 -> Delay2/1
  Delay9/1 -> Add4/2

== system coif2_7_Level/3rd_Level_Decomp/HiD_Odd ==
  In_HiD_o : Inport  OutDataTypeStr=double  SampleTime=1/44100
  Add{,1..4} (5 alike) : Sum  AccumDataTypeStr=double  OutDataTypeStr=double
  Delay{,1..9} (10 alike) : Delay  DelayLength=1  SampleTime=1/44100
  HiD_1 : Constant  Value=-0.041464937  OutDataTypeStr=double  SampleTime=1/44100
  HiD_11 : Constant  Value=-0.000720549  OutDataTypeStr=double  SampleTime=1/44100
  HiD_3 : Constant  Value=0.386110067  OutDataTypeStr=double  SampleTime=1/44100
  HiD_5 : Constant  Value=0.417005184  OutDataTypeStr=double  SampleTime=1/44100
  HiD_7 : Constant  Value=-0.059434419  OutDataTypeStr=double  SampleTime=1/44100
  HiD_9 : Constant  Value=0.005611435  OutDataTypeStr=double  SampleTime=1/44100
  Multiply{,1..5} (6 alike) : Product  OutDataTypeStr=double
  Rate Transition{,1..4} (5 alike) : RateTransition  OutPortSampleTime=1/44100
  Out_HiD_o : Outport  OutDataTypeStr=double  SampleTime=1/44100  VectorParamsAs1DForOutWhenUnconnected=off
  wires:
  Add/1 -> Out_HiD_o/1
  Add4/1 -> Delay2/1
  Delay8/1 -> Rate Transition4/1
  Rate Transition4/1 -> Multiply3/2, Delay4/1
  HiD_7/1 -> Multiply3/1
  Add2/1 -> Delay9/1
  Delay1/1 -> Rate Transition1/1
  Delay2/1 -> Add1/2
  Delay6/1 -> Add3/2
  HiD_9/1 -> Multiply4/1
  Add3/1 -> Delay7/1
  Multiply3/1 -> Add2/1
  Multiply5/1 -> Delay6/1
  Delay7/1 -> Add2/2
  HiD_3/1 -> Multiply1/1
  Multiply4/1 -> Add3/1
  Rate Transition3/1 -> Multiply5/2
  HiD_1/1 -> Multiply/1
  HiD_11/1 -> Multiply5/1
  Delay4/1 -> Rate Transition2/1
  Rate Transition2/1 -> Delay5/1, Multiply4/2
  Multiply2/1 -> Add4/1
  Delay/1 -> Rate Transition/1
  Rate Transition/1 -> Delay1/1, Multiply1/2
  Delay5/1 -> Rate Transition3/1
  Delay9/1 -> Add4/2
  Multiply1/1 -> Add1/1
  Rate Transition1/1 -> Delay8/1, Multiply2/2
  Multiply/1 -> Add/1
  Add1/1 -> Delay3/1
  Delay3/1 -> Add/2
  In_HiD_o/1 -> Delay/1, Multiply/2
  HiD_5/1 -> Multiply2/1

== system coif2_7_Level/3rd_Level_Decomp/LoD_Even ==
  In_LoD_e : Inport  OutDataTypeStr=double  SampleTime=1/44100
  Add{,1..4} (5 alike) : Sum  AccumDataTypeStr=double  OutDataTypeStr=double
  Delay{,1..9} (10 alike) : Delay  DelayLength=1  SampleTime=1/44100
  LoD_0 : Constant  Value=-0.000720549  OutDataTypeStr=double  SampleTime=1/44100
  LoD_10 : Constant  Value=-0.041464937  OutDataTypeStr=double  SampleTime=1/44100
  LoD_2 : Constant  Value=0.005611435  OutDataTypeStr=double  SampleTime=1/44100
  LoD_4 : Constant  Value=-0.059434419  OutDataTypeStr=double  SampleTime=1/44100
  LoD_6 : Constant  Value=0.417005184  OutDataTypeStr=double  SampleTime=1/44100
  LoD_8 : Constant  Value=0.386110067  OutDataTypeStr=double  SampleTime=1/44100
  Multiply{,1..5} (6 alike) : Product  OutDataTypeStr=double
  Rate Transition{,1..4} (5 alike) : RateTransition  OutPortSampleTime=1/44100
  Out_LoD_e : Outport  OutDataTypeStr=double  SampleTime=1/44100  VectorParamsAs1DForOutWhenUnconnected=off
  wires:
  Delay3/1 -> Add/2
  Rate Transition1/1 -> Delay8/1, Multiply2/2
  Add/1 -> Out_LoD_e/1
  Add1/1 -> Delay3/1
  Multiply/1 -> Add/1
  In_LoD_e/1 -> Delay/1, Multiply/2
  Rate Transition/1 -> Delay1/1, Multiply1/2
  LoD_4/1 -> Multiply2/1
  Delay/1 -> Rate Transition/1
  Delay9/1 -> Add4/2
  Multiply1/1 -> Add1/1
  Multiply2/1 -> Add4/1
  LoD_2/1 -> Multiply1/1
  Delay4/1 -> Rate Transition2/1
  Multiply5/1 -> Delay6/1
  Multiply4/1 -> Add3/1
  Rate Transition2/1 -> Delay5/1, Multiply4/2
  LoD_10/1 -> Multiply5/1
  Delay2/1 -> Add1/2
  Delay5/1 -> Rate Transition3/1
  Multiply3/1 -> Add2/1
  LoD_8/1 -> Multiply4/1
  Delay7/1 -> Add2/2
  Rate Transition3/1 -> Multiply5/2
  Delay6/1 -> Add3/2
  Add3/1 -> Delay7/1
  LoD_6/1 -> Multiply3/1
  LoD_0/1 -> Multiply/1
  Add2/1 -> Delay9/1
  Delay8/1 -> Rate Transition4/1
  Rate Transition4/1 -> Multiply3/2, Delay4/1
  Delay1/1 -> Rate Transition1/1
  Add4/1 -> Delay2/1

== system coif2_7_Level/3rd_Level_Decomp/LoD_Odd ==
  In_LoD_o : Inport  OutDataTypeStr=double  SampleTime=1/44100
  Add{,1..4} (5 alike) : Sum  AccumDataTypeStr=double  OutDataTypeStr=double
  Delay{,1..9} (10 alike) : Delay  DelayLength=1  SampleTime=1/44100
  LoD_{1,5,7,11} (4 alike) : Constant  Value=-0.07273262  OutDataTypeStr=double  SampleTime=1/44100
  LoD_3 : Constant  Value=0.85257202  OutDataTypeStr=double  SampleTime=1/44100
  LoD_9 : Constant  Value=0.85257202  OutDataTypeStr=double  SampleTime=1/44100
  Multiply{,1..5} (6 alike) : Product  OutDataTypeStr=double
  Rate Transition{,1..4} (5 alike) : RateTransition  OutPortSampleTime=1/44100
  Out_LoD_o : Outport  OutDataTypeStr=double  SampleTime=1/44100  VectorParamsAs1DForOutWhenUnconnected=off
  wires:
  LoD_9/1 -> Multiply4/1
  Add3/1 -> Delay7/1
  Rate Transition4/1 -> Multiply3/2, Delay4/1
  Delay2/1 -> Add1/2
  Delay1/1 -> Rate Transition1/1
  Delay8/1 -> Rate Transition4/1
  LoD_5/1 -> Multiply2/1
  Add4/1 -> Delay2/1
  LoD_11/1 -> Multiply5/1
  LoD_1/1 -> Multiply/1
  Multiply3/1 -> Add2/1
  LoD_3/1 -> Multiply1/1
  In_LoD_o/1 -> Delay/1, Multiply/2
  Add/1 -> Out_LoD_o/1
  Rate Transition1/1 -> Delay8/1, Multiply2/2
  Multiply1/1 -> Add1/1
  Delay/1 -> Rate Transition/1
  Rate Transition/1 -> Delay1/1, Multiply1/2
  Multiply2/1 -> Add4/1
  LoD_7/1 -> Multiply3/1
  Rate Transition2/1 -> Delay5/1, Multiply4/2
  Delay4/1 -> Rate Transition2/1
  Multiply5/1 -> Delay6/1
  Delay7/1 -> Add2/2
  Rate Transition3/1 -> Multiply5/2
  Delay3/1 -> Add/2
  Delay5/1 -> Rate Transition3/1
  Add2/1 -> Delay9/1
  Add1/1 -> Delay3/1
  Delay9/1 -> Add4/2
  Delay6/1 -> Add3/2
  Multiply4/1 -> Add3/1
  Multiply/1 -> Add/1

== system coif2_7_Level/3rd_Level_Recon/HiR_Even ==
  In_HiR_e : Inport  OutDataTypeStr=double  SampleTime=1/44100
  Add{,1..4} (5 alike) : Sum  AccumDataTypeStr=double  OutDataTypeStr=double
  Delay{,1..9} (10 alike) : Delay  DelayLength=1  SampleTime=1/44100
  HiR_0 : Constant  Value=-0.000720549  OutDataTypeStr=double  SampleTime=1/44100
  HiR_10 : Constant  Value=-0.041464937  OutDataTypeStr=double  SampleTime=1/44100
  HiR_2 : Constant  Value=0.005611435  OutDataTypeStr=double  SampleTime=1/44100
  HiR_4 : Constant  Value=-0.059434419  OutDataTypeStr=double  SampleTime=1/44100
  HiR_6 : Constant  Value=0.417005184  OutDataTypeStr=double  SampleTime=1/44100
  HiR_8 : Constant  Value=0.386110067  OutDataTypeStr=double  SampleTime=1/44100
  Multiply{,1..5} (6 alike) : Product  OutDataTypeStr=double
  Rate Transition{,1..4} (5 alike) : RateTransition  OutPortSampleTime=1/44100
  Out_HiR_e : Outport  OutDataTypeStr=double  SampleTime=1/44100  VectorParamsAs1DForOutWhenUnconnected=off
  wires:
  Multiply1/1 -> Add1/1
  Delay4/1 -> Rate Transition2/1
  Add4/1 -> Delay2/1
  Delay9/1 -> Add4/2
  Rate Transition4/1 -> Multiply3/2, Delay4/1
  Rate Transition3/1 -> Multiply5/2
  Add1/1 -> Delay3/1
  Add3/1 -> Delay7/1
  Delay8/1 -> Rate Transition4/1
  Multiply5/1 -> Delay6/1
  Add2/1 -> Delay9/1
  Multiply4/1 -> Add3/1
  HiR_8/1 -> Multiply4/1
  Delay6/1 -> Add3/2
  Rate Transition1/1 -> Delay8/1, Multiply2/2
  In_HiR_e/1 -> Delay/1, Multiply/2
  HiR_0/1 -> Multiply/1
  Multiply2/1 -> Add4/1
  Delay7/1 -> Add2/2
  Rate Transition2/1 -> Delay5/1, Multiply4/2
  Add/1 -> Out_HiR_e/1
  Multiply3/1 -> Add2/1
  HiR_6/1 -> Multiply3/1
  Multiply/1 -> Add/1
  HiR_4/1 -> Multiply2/1
  Delay2/1 -> Add1/2
  Delay5/1 -> Rate Transition3/1
  Delay3/1 -> Add/2
  Delay1/1 -> Rate Transition1/1
  HiR_2/1 -> Multiply1/1
  Rate Transition/1 -> Delay1/1, Multiply1/2
  Delay/1 -> Rate Transition/1
  HiR_10/1 -> Multiply5/1

== system coif2_7_Level/3rd_Level_Recon/HiR_Odd ==
  In_HiR_o : Inport  OutDataTypeStr=double  SampleTime=1/44100
  Add{,1..4} (5 alike) : Sum  AccumDataTypeStr=double  OutDataTypeStr=double
  Delay{,1..9} (10 alike) : Delay  DelayLength=1  SampleTime=1/44100
  HiR_1 : Constant  Value=0.001823209  OutDataTypeStr=double  SampleTime=1/44100
  HiR_11 : Constant  Value=-0.016387336  OutDataTypeStr=double  SampleTime=1/44100
  HiR_3 : Constant  Value=-0.023680172  OutDataTypeStr=double  SampleTime=1/44100
  HiR_5 : Constant  Value=0.076488599  OutDataTypeStr=double  SampleTime=1/44100
  HiR_7 : Constant  Value=-0.812723635  OutDataTypeStr=double  SampleTime=1/44100
  HiR_9 : Constant  Value=0.067372555  OutDataTypeStr=double  SampleTime=1/44100
  Multiply{,1..5} (6 alike) : Product  OutDataTypeStr=double
  Rate Transition{,1..4} (5 alike) : RateTransition  OutPortSampleTime=1/44100
  Out_HiR_o : Outport  OutDataTypeStr=double  SampleTime=1/44100  VectorParamsAs1DForOutWhenUnconnected=off
  wires:
  HiR_9/1 -> Multiply4/1
  Add2/1 -> Delay9/1
  Rate Transition/1 -> Delay1/1, Multiply1/2
  HiR_7/1 -> Multiply3/1
  Multiply2/1 -> Add4/1
  Rate Transition2/1 -> Delay5/1, Multiply4/2
  Rate Transition4/1 -> Multiply3/2, Delay4/1
  HiR_5/1 -> Multiply2/1
  Multiply5/1 -> Delay6/1
  HiR_11/1 -> Multiply5/1
  Multiply1/1 -> Add1/1
  Delay5/1 -> Rate Transition3/1
  Add1/1 -> Delay3/1
  Multiply/1 -> Add/1
  Delay7/1 -> Add2/2
  Delay2/1 -> Add1/2
  Delay9/1 -> Add4/2
  Delay4/1 -> Rate Transition2/1
  Delay3/1 -> Add/2
  Multiply3/1 -> Add2/1
  Delay8/1 -> Rate Transition4/1
  Rate Transition3/1 -> Multiply5/2
  Delay1/1 -> Rate Transition1/1
  Delay6/1 -> Add3/2
  Add4/1 -> Delay2/1
  Rate Transition1/1 -> Delay8/1, Multiply2/2
  Add/1 -> Out_HiR_o/1
  Add3/1 -> Delay7/1
  HiR_3/1 -> Multiply1/1
  In_HiR_o/1 -> Multiply/2, Delay/1
  Delay/1 -> Rate Transition/1
  HiR_1/1 -> Multiply/1
  Multiply4/1 -> Add3/1

== system coif2_7_Level/3rd_Level_Recon/LoR_Even ==
  In_LoR_e : Inport  OutDataTypeStr=double  SampleTime=1/44100
  Add{,1..4} (5 alike) : Sum  AccumDataTypeStr=double  OutDataTypeStr=double
  Delay{,1..9} (10 alike) : Delay  DelayLength=1  SampleTime=1/44100
  LoR_0 : Constant  Value=0.016387336  OutDataTypeStr=double  SampleTime=1/44100
  LoR_10 : Constant  Value=-0.001823209  OutDataTypeStr=double  SampleTime=1/44100
  LoR_2 : Constant  Value=-0.067372555  OutDataTypeStr=double  SampleTime=1/44100
  LoR_4 : Constant  Value=0.812723635  OutDataTypeStr=double  SampleTime=1/44100
  LoR_6 : Constant  Value=-0.076488599  OutDataTypeStr=double  SampleTime=1/44100
  LoR_8 : Constant  Value=0.023680172  OutDataTypeStr=double  SampleTime=1/44100
  Multiply{,1..5} (6 alike) : Product  OutDataTypeStr=double
  Rate Transition{,1..4} (5 alike) : RateTransition  OutPortSampleTime=1/44100
  Out_LoR_e : Outport  OutDataTypeStr=double  SampleTime=1/44100  VectorParamsAs1DForOutWhenUnconnected=off
  wires:
  LoR_4/1 -> Multiply2/1
  LoR_10/1 -> Multiply5/1
  LoR_8/1 -> Multiply4/1
  LoR_0/1 -> Multiply/1
  LoR_2/1 -> Multiply1/1
  Add2/1 -> Delay9/1
  In_LoR_e/1 -> Multiply/2, Delay/1
  Multiply4/1 -> Add3/1
  Delay8/1 -> Rate Transition4/1
  Add3/1 -> Delay7/1
  Rate Transition3/1 -> Multiply5/2
  Add4/1 -> Delay2/1
  Delay4/1 -> Rate Transition2/1
  Multiply1/1 -> Add1/1
  Delay5/1 -> Rate Transition3/1
  Delay2/1 -> Add1/2
  Delay3/1 -> Add/2
  Delay1/1 -> Rate Transition1/1
  Multiply/1 -> Add/1
  Multiply3/1 -> Add2/1
  Delay9/1 -> Add4/2
  Rate Transition2/1 -> Delay5/1, Multiply4/2
  Rate Transition4/1 -> Multiply3/2, Delay4/1
  Add1/1 -> Delay3/1
  LoR_6/1 -> Multiply3/1
  Multiply5/1 -> Delay6/1
  Add/1 -> Out_LoR_e/1
  Rate Transition1/1 -> Delay8/1, Multiply2/2
  Delay6/1 -> Add3/2
  Multiply2/1 -> Add4/1
  Delay7/1 -> Add2/2
  Rate Transition/1 -> Delay1/1, Multiply1/2
  Delay/1 -> Rate Transition/1

== system coif2_7_Level/3rd_Level_Recon/LoR_Odd ==
  In_LoR_o : Inport  OutDataTypeStr=double  SampleTime=1/44100
  Add{,1..4} (5 alike) : Sum  AccumDataTypeStr=double  OutDataTypeStr=double
  Delay{,1..9} (10 alike) : Delay  DelayLength=1  SampleTime=1/44100
  LoR_1 : Constant  Value=-0.041464937  OutDataTypeStr=double  SampleTime=1/44100
  LoR_11 : Constant  Value=-0.000720549  OutDataTypeStr=double  SampleTime=1/44100
  LoR_3 : Constant  Value=0.386110067  OutDataTypeStr=double  SampleTime=1/44100
  LoR_5 : Constant  Value=0.417005184  OutDataTypeStr=double  SampleTime=1/44100
  LoR_7 : Constant  Value=-0.059434419  OutDataTypeStr=double  SampleTime=1/44100
  LoR_9 : Constant  Value=0.005611435  OutDataTypeStr=double  SampleTime=1/44100
  Multiply{,1..5} (6 alike) : Product  OutDataTypeStr=double
  Rate Transition{,1..4} (5 alike) : RateTransition  OutPortSampleTime=1/44100
  Out_HiR_o : Outport  OutDataTypeStr=double  SampleTime=1/44100  VectorParamsAs1DForOutWhenUnconnected=off
  wires:
  LoR_9/1 -> Multiply4/1
  Add2/1 -> Delay9/1
  Rate Transition/1 -> Delay1/1, Multiply1/2
  LoR_7/1 -> Multiply3/1
  Multiply2/1 -> Add4/1
  Rate Transition2/1 -> Delay5/1, Multiply4/2
  Rate Transition4/1 -> Multiply3/2, Delay4/1
  LoR_5/1 -> Multiply2/1
  Multiply5/1 -> Delay6/1
  LoR_11/1 -> Multiply5/1
  Multiply1/1 -> Add1/1
  Delay5/1 -> Rate Transition3/1
  Add1/1 -> Delay3/1
  Multiply/1 -> Add/1
  Delay7/1 -> Add2/2
  Delay2/1 -> Add1/2
  Delay9/1 -> Add4/2
  Delay4/1 -> Rate Transition2/1
  Delay3/1 -> Add/2
  Multiply3/1 -> Add2/1
  Delay8/1 -> Rate Transition4/1
  Rate Transition3/1 -> Multiply5/2
  Delay1/1 -> Rate Transition1/1
  Delay6/1 -> Add3/2
  Add4/1 -> Delay2/1
  Rate Transition1/1 -> Delay8/1, Multiply2/2
  Add/1 -> Out_HiR_o/1
  Add3/1 -> Delay7/1
  LoR_3/1 -> Multiply1/1
  In_LoR_o/1 -> Multiply/2, Delay/1
  Delay/1 -> Rate Transition/1
  LoR_1/1 -> Multiply/1
  Multiply4/1 -> Add3/1

== system coif2_7_Level/4th_Level_Decomp/HiD_Even ==
  In_HiD_e : Inport  OutDataTypeStr=double  SampleTime=1/44100
  Add{,1..4} (5 alike) : Sum  AccumDataTypeStr=double  OutDataTypeStr=double
  Delay{,1..9} (10 alike) : Delay  DelayLength=1  SampleTime=1/44100
  HiD_0 : Constant  Value=-0.016387336  OutDataTypeStr=double  SampleTime=1/44100
  HiD_10 : Constant  Value=0.001823209  OutDataTypeStr=double  SampleTime=1/44100
  HiD_2 : Constant  Value=0.067372555  OutDataTypeStr=double  SampleTime=1/44100
  HiD_4 : Constant  Value=-0.812723635  OutDataTypeStr=double  SampleTime=1/44100
  HiD_6 : Constant  Value=0.076488599  OutDataTypeStr=double  SampleTime=1/44100
  HiD_8 : Constant  Value=-0.023680172  OutDataTypeStr=double  SampleTime=1/44100
  Multiply{,1..5} (6 alike) : Product  OutDataTypeStr=double
  Rate Transition{,1..4} (5 alike) : RateTransition  OutPortSampleTime=1/44100
  Out_HiD_e : Outport  OutDataTypeStr=double  SampleTime=1/44100  VectorParamsAs1DForOutWhenUnconnected=off
  wires:
  In_HiD_e/1 -> Delay/1, Multiply/2
  Delay3/1 -> Add/2
  HiD_2/1 -> Multiply1/1
  Delay/1 -> Rate Transition/1
  Multiply/1 -> Add/1
  Rate Transition/1 -> Delay1/1, Multiply1/2
  HiD_4/1 -> Multiply2/1
  Delay2/1 -> Add1/2
  Multiply1/1 -> Add1/1
  Add1/1 -> Delay3/1
  Rate Transition1/1 -> Delay8/1, Multiply2/2
  Add/1 -> Out_HiD_e/1
  Delay1/1 -> Rate Transition1/1
  HiD_0/1 -> Multiply/1
  HiD_6/1 -> Multiply3/1
  Delay7/1 -> Add2/2
  Delay5/1 -> Rate Transition3/1
  Rate Transition3/1 -> Multiply5/2
  Add3/1 -> Delay7/1
  Multiply3/1 -> Add2/1
  Rate Transition2/1 -> Delay5/1, Multiply4/2
  Delay6/1 -> Add3/2
  Multiply4/1 -> Add3/1
  Multiply5/1 -> Delay6/1
  HiD_10/1 -> Multiply5/1
  Delay4/1 -> Rate Transition2/1
  HiD_8/1 -> Multiply4/1
  Delay8/1 -> Rate Transition4/1
  Rate Transition4/1 -> Multiply3/2, Delay4/1
  Add2/1 -> Delay9/1
  Multiply2/1 -> Add4/1
  Add4/1 -> Delay2/1
  Delay9/1 -> Add4/2
